simulink model "generic_truck"  (R2025a)
settings: Solver=VariableStepAuto  StartTime=0.0  StopTime=600  FixedStep=0.01  MaxStep=0.001  RelTol=1e-3  EnableMultiTasking=on
libraries: TruckMaker4SL x205, simulink x1
(part 7 of 9)

== matlab function generic_truck/TruckMaker/Subsystem1/ONE_TRACK_MODEL_TRACTOR_UKF/Working Model with 7 measurements ==
  data: z input; u input; xhat output; Q input; R input; Ts input; P output; dxdt output; innovation output; K_out output; S_out output; z_pred_out output; data input
function [xhat, P, dxdt, innovation, K_out, S_out, z_pred_out] = UKF_OneTrack_IMU(z, u, Q, R, Ts,data)

persistent x Pk dxdt_old t p_nom Pp

if isempty(x)
    x = [15;0.1;0.1;7.5;7.5];
end
if isempty(Pk)
    Pk = diag([0.1 0.1 0.1 5 5]);
end
if isempty(dxdt_old)
    dxdt_old = zeros(5,1);
end
if isempty(t)
    t = 0;
end
if isempty(p_nom)
    p_nom = [6800; 12994.917];
    Pp = diag([5000, 20000]).^2;
end

T_sim = 0.001;
t = t + T_sim;
t=data;

if t < 30
    xhat = x;
    P = Pk;
    dxdt = dxdt_old;
    innovation = zeros(length(z),1);
    K_out = zeros(length(x), length(z));
    S_out = eye(length(z));
    z_pred_out = zeros(length(z),1);
    return
end

IDX_VX  = 3; 
IDX_WRL = 6; 
IDX_WRR = 7;

g  = 9.82;

p_cog = [3.473;0;0.925];
p_fax = [4.520;0;0.490];
p_rax = [0.950;0;0.490];
p_imu = [3.600;0;1.000];

lf = abs(p_fax(1)-p_cog(1));
lr = abs(p_cog(1)-p_rax(1));
L  = lf + lr;
h  = p_cog(3);

Rfax = p_fax - p_cog; Rfax(3) = -p_cog(3);
Rrax = p_rax - p_cog; Rrax(3) = -p_cog(3);
Rcog = p_imu - p_cog;

delta = u(1);
T_rl  = u(2);
T_rr  = u(3);
Rwheel = 0.505;
Fx_vehicle = (T_rl + T_rr)/Rwheel;

n  = length(x);
np = length(p_nom);
nSPx = 2*n + 1;
nSPp = 2*np;
nSP  = nSPx + nSPp;

W0 = 1 - (n + np)/3;
Wi = (1 - W0)/(2*(n + np));
gamma = sqrt((n + np)/(1 - W0));

%% ===== STATE SIGMA =====
Pk = (Pk + Pk')/2 + 1e-9*eye(n);
Sx = chol(Pk,'lower');

X = zeros(n,nSPx);
X(:,1) = x;
for i=1:n
    X(:,i+1)   = x + gamma*Sx(:,i);
    X(:,i+1+n) = x - gamma*Sx(:,i);
end

%% ===== PARAM SIGMA =====
Pp = (Pp + Pp')/2 + 1e-9*eye(np);
Sp = chol(Pp,'lower');

SPp = zeros(np,nSPp);
for i=1:np
    SPp(:,i)    = p_nom + gamma*Sp(:,i);
    SPp(:,i+np) = p_nom - gamma*Sp(:,i);
end

%% ===== PREDICTION =====
X_prop = zeros(n,nSP);
dxdt_model = zeros(5,1);

for k=1:nSP
    if k <= nSPx
        Xk = X(:,k); 
        pk = p_nom;
    else
        Xk = x; 
        pk = SPp(:,k-nSPx);
    end

    vx=Xk(1); vy=Xk(2); wz=Xk(3); Cf=Xk(4); Cr=Xk(5);
    m=pk(1); Jz=pk(2);

    v_cog=[vx;vy;0]; omega=[0;0;wz];
    Rotf=[cos(delta) -sin(delta) 0; sin(delta) cos(delta) 0; 0 0 1];

    vf=Rotf.'*(v_cog+cross(omega,Rfax));
    vr=v_cog+cross(omega,Rrax);

    alpha_f=atan2(vf(2),max(abs(vf(1)),0.1));
    alpha_r=atan2(vr(2),max(abs(vr(1)),0.1));

    ax_est=Fx_vehicle/m+vy*wz;

    Ffz=m*g*lr/L - m*ax_est*h/L;
    Frz=m*g*lf/L + m*ax_est*h/L;

    Fy_f=-Cf*alpha_f*Ffz;
    Fy_r=-Cr*alpha_r*Frz;

    dvx=(Fx_vehicle - Fy_f*sin(delta))/m + vy*wz;
    dvy=(Fy_f*cos(delta)+Fy_r)/m - vx*wz;
    dwz=(lf*Fy_f*cos(delta) - lr*Fy_r)/Jz;

    if k==1
        dxdt_model=[dvx;dvy;dwz;0;0];
    end

    X_prop(:,k)=[vx+Ts*dvx; vy+Ts*dvy; wz+Ts*dwz; Cf; Cr];
end

%% ===== MEAN =====
x_pred=zeros(n,1);
for k=1:nSP
    w=(k==1)*W0 + (k>1)*Wi;
    x_pred=x_pred + w*X_prop(:,k);
end

%% ===== COV =====
P_pred=zeros(n);
for k=1:nSPx
    w=(k==1)*W0 + (k>1)*Wi;
    dx=X_prop(:,k)-x_pred;
    P_pred=P_pred + w*(dx*dx');
end
P_pred=P_pred + Q*Ts;

%% ===== NEW SIGMA POINTS =====
P_pred=(P_pred+P_pred')/2 + 1e-9*eye(n);
Sx=chol(P_pred,'lower');

SPx_new=zeros(n,nSPx);
SPx_new(:,1)=x_pred;

for i=1:n
    SPx_new(:,i+1)=x_pred+gamma*Sx(:,i);
    SPx_new(:,i+1+n)=x_pred-gamma*Sx(:,i);
end

%% ===== MEASUREMENT =====
Z=zeros(length(z),nSP);

for k=1:nSP
    if k<=nSPx
        Xk=SPx_new(:,k);
        pk=p_nom;
    else
        Xk=x_pred;
        pk=SPp(:,k-nSPx);
    end

    vx=Xk(1); vy=Xk(2); wz=Xk(3);
    Cf=Xk(4); Cr=Xk(5);

    m=pk(1); Jz=pk(2);

    v_cog=[vx;vy;0]; omega=[0;0;wz];
    Rotf=[cos(delta) -sin(delta) 0; sin(delta) cos(delta) 0; 0 0 1];

    vf=Rotf.'*(v_cog+cross(omega,Rfax));
    vr=v_cog+cross(omega,Rrax);

    alpha_f=atan2(vf(2),max(abs(vf(1)),0.1));
    alpha_r=atan2(vr(2),max(abs(vr(1)),0.1));

    ax_est=Fx_vehicle/m+vy*wz;

    Ffz=m*g*lr/L - m*ax_est*h/L;
    Frz=m*g*lf/L + m*ax_est*h/L;

    Fy_f=-Cf*alpha_f*Ffz;
    Fy_r=-Cr*alpha_r*Frz;

    dvx=(Fx_vehicle - Fy_f*sin(delta))/m;
    dvy=(Fy_f*cos(delta)+Fy_r)/m;
    dwz=(lf*Fy_f*cos(delta) - lr*Fy_r)/Jz;

    a_cog=[dvx;dvy;0];
    alpha_vec=[0;0;dwz];

    a_imu=a_cog + cross(omega,cross(omega,Rcog)) + cross(alpha_vec,Rcog);
    v_imu=v_cog + cross(omega,Rcog);

    omega_rl=vx/Rwheel;
    omega_rr=vx/Rwheel;

    Z(:,k)=[a_imu(1:2); v_imu(1:2); wz; omega_rl; omega_rr];
end

%% ===== z mean =====
z_pred=zeros(length(z),1);
for k=1:nSP
    w=(k==1)*W0 + (k>1)*Wi;
    z_pred=z_pred + w*Z(:,k);
end

%% ===== SENSOR SELECTION =====
valid_idx=true(length(z),1);

if ~isnan(z(IDX_VX))
    valid_idx(IDX_WRL)=false;
    valid_idx(IDX_WRR)=false;
else
    valid_idx(IDX_VX)=false;
end

valid_idx=valid_idx & ~isnan(z);

z_used=z(valid_idx);
z_pred_used=z_pred(valid_idx);
Z_used=Z(valid_idx,:);
R_used=R(valid_idx,valid_idx);

%% ===== S =====
S_cov=zeros(length(z_used));
for k=1:nSP
    w=(k==1)*W0 + (k>1)*Wi;
    dz=Z_used(:,k)-z_pred_used;
    S_cov=S_cov + w*(dz*dz');
end

S_cov=S_cov + R_used;
S_cov=(S_cov+S_cov')/2 + 1e-9*eye(size(S_cov));

%% ===== Pxz =====
Pxz=zeros(n,length(z_used));
for k=1:nSPx
    w=(k==1)*W0 + (k>1)*Wi;
    dx=SPx_new(:,k)-x_pred;
    dz=Z_used(:,k)-z_pred_used;
    Pxz=Pxz + w*(dx*dz');
end

%% ===== UPDATE =====
K=Pxz/S_cov;

x=x_pred + K*(z_used - z_pred_used);
Pk=P_pred - K*S_cov*K';
Pk=(Pk+Pk')/2 + 1e-9*eye(n);

%% ===== OUTPUT =====
xhat=x;
P=Pk;
dxdt=dxdt_model;

innovation=zeros(length(z),1);
innovation(valid_idx)=z_used - z_pred_used;

K_out=zeros(n,length(z));
K_out(:,valid_idx)=K;

S_out=zeros(length(z));
S_out(valid_idx,valid_idx)=S_cov;

z_pred_out=z_pred;

end

== matlab function generic_truck/TruckMaker/Subsystem1/ONE_TRACK_MODEL_TRACTOR_UKF/MATLAB Function1 ==
  data: z input; u input; xhat output; Q input; R input; Ts input; data input; P output; dxdt output; innovation output; K_out output; S_out output; z_pred_out output
function [xhat, P, dxdt, innovation, K_out, S_out, z_pred_out] = UKF_OneTrack_IMU(z, u, Q, R, Ts,data)

persistent x Pk dxdt_old t p_nom Pp

if isempty(x)
    x = [15;0.1;0.1;7.5;7.5];
end
if isempty(Pk)
    Pk = diag([0.1 0.1 0.1 5 5]);
end
if isempty(dxdt_old)
    dxdt_old = zeros(5,1);
end
if isempty(t)
    t = 0;
end
if isempty(p_nom)
    p_nom = [6800; 12994.917];
    Pp = diag([5000, 20000]).^2;
end

T_sim = 0.001;
t = t + T_sim;
t=data;

if t < 30
    xhat = x;
    P = Pk;
    dxdt = dxdt_old;
    innovation = zeros(length(z),1);
    K_out = zeros(length(x), length(z));
    S_out = eye(length(z));
    z_pred_out = zeros(length(z),1);
    return
end

IDX_VX  = 3; 
IDX_WRL = 6; 
IDX_WRR = 7;

g  = 9.82;

p_cog = [3.473;0;0.925];
p_fax = [4.520;0;0.490];
p_rax = [0.950;0;0.490];
p_imu = [3.600;0;1.000];

lf = abs(p_fax(1)-p_cog(1));
lr = abs(p_cog(1)-p_rax(1));
L  = lf + lr;
h  = p_cog(3);

Rfax = p_fax - p_cog; Rfax(3) = -p_cog(3);
Rrax = p_rax - p_cog; Rrax(3) = -p_cog(3);
Rcog = p_imu - p_cog;

delta = u(1);
T_rl  = u(2);
T_rr  = u(3);
Rwheel = 0.505;
Fx_vehicle = (T_rl + T_rr)/Rwheel;

n  = length(x);
np = length(p_nom);
nSPx = 2*n + 1;
nSPp = 2*np;
nSP  = nSPx + nSPp;

W0 = 1 - (n + np)/3;
Wi = (1 - W0)/(2*(n + np));
gamma = sqrt((n + np)/(1 - W0));

%% ===== STATE SIGMA =====
Pk = (Pk + Pk')/2 + 1e-9*eye(n);
Sx = chol(Pk,'lower');

X = zeros(n,nSPx);
X(:,1) = x;
for i=1:n
    X(:,i+1)   = x + gamma*Sx(:,i);
    X(:,i+1+n) = x - gamma*Sx(:,i);
end

%% ===== PARAM SIGMA =====
Pp = (Pp + Pp')/2 + 1e-9*eye(np);
Sp = chol(Pp,'lower');

SPp = zeros(np,nSPp);
for i=1:np
    SPp(:,i)    = p_nom + gamma*Sp(:,i);
    SPp(:,i+np) = p_nom - gamma*Sp(:,i);
end

%% ===== PREDICTION =====
X_prop = zeros(n,nSP);
dxdt_model = zeros(5,1);

for k=1:nSP
    if k <= nSPx
        Xk = X(:,k); 
        pk = p_nom;
    else
        Xk = x; 
        pk = SPp(:,k-nSPx);
    end

    vx=Xk(1); vy=Xk(2); wz=Xk(3); Cf=Xk(4); Cr=Xk(5);
    m=pk(1); Jz=pk(2);

    v_cog=[vx;vy;0]; 
    omega=[0;0;wz];

    Rotf=[cos(delta) -sin(delta) 0;
          sin(delta)  cos(delta)  0; 
           0          0          1];

    vf=Rotf.'*(v_cog+cross(omega,Rfax));
    vr=v_cog+cross(omega,Rrax);

    alpha_f=atan2(vf(2),max(abs(vf(1)),0.1));
    alpha_r=atan2(vr(2),max(abs(vr(1)),0.1));

    ax_est=Fx_vehicle/m+vy*wz;

    Ffz=m*g*lr/L - m*ax_est*h/L;
    Frz=m*g*lf/L + m*ax_est*h/L;

    Fy_f=-Cf*alpha_f*Ffz;
    Fy_r=-Cr*alpha_r*Frz;

    dvx=(Fx_vehicle - Fy_f*sin(delta))/m + vy*wz;
    dvy=(Fy_f*cos(delta)+Fy_r)/m - vx*wz;
    dwz=(lf*Fy_f*cos(delta) - lr*Fy_r)/Jz;

    if k==1
        dxdt_model=[dvx;dvy;dwz;0;0];
    end

    X_prop(:,k)=[vx+Ts*dvx; vy+Ts*dvy; wz+Ts*dwz; Cf; Cr];
end

%% ===== MEAN =====
x_pred=zeros(n,1);
for k=1:nSP
    w=(k==1)*W0 + (k>1)*Wi;
    x_pred=x_pred + w*X_prop(:,k);
end

%% ===== COV =====
P_pred=zeros(n);
for k=1:nSPx
    w=(k==1)*W0 + (k>1)*Wi;
    dx=X_prop(:,k)-x_pred;
    P_pred=P_pred + w*(dx*dx');
end
P_pred=P_pred + Q*Ts;

%% ===== NEW SIGMA POINTS =====
P_pred=(P_pred+P_pred')/2 + 1e-9*eye(n);
Sx=chol(P_pred,'lower');

SPx_new=zeros(n,nSPx);
SPx_new(:,1)=x_pred;

for i=1:n
    SPx_new(:,i+1)  =x_pred+gamma*Sx(:,i);
    SPx_new(:,i+1+n) =x_pred-gamma*Sx(:,i);
end

%% ===== MEASUREMENT =====
Z=zeros(length(z),nSP);

for k=1:nSP
    if k<=nSPx
        Xk=SPx_new(:,k);
        pk=p_nom;
    else
        Xk=x_pred;
        pk=SPp(:,k-nSPx);
    end

    vx=Xk(1); vy=Xk(2); wz=Xk(3);
    Cf=Xk(4); Cr=Xk(5);

    m=pk(1); Jz=pk(2);

    v_cog=[vx;vy;0]; omega=[0;0;wz];
    Rotf=[cos(delta) -sin(delta) 0; sin(delta) cos(delta) 0; 0 0 1];

    vf=Rotf.'*(v_cog+cross(omega,Rfax));
    vr=v_cog+cross(omega,Rrax);

    alpha_f=atan2(vf(2),max(abs(vf(1)),0.1));
    alpha_r=atan2(vr(2),max(abs(vr(1)),0.1));

    ax_est=Fx_vehicle/m+vy*wz;

    Ffz=m*g*lr/L - m*ax_est*h/L;
    Frz=m*g*lf/L + m*ax_est*h/L;

    Fy_f=-Cf*alpha_f*Ffz;
    Fy_r=-Cr*alpha_r*Frz;

    dvx=(Fx_vehicle - Fy_f*sin(delta))/m;
    dvy=(Fy_f*cos(delta)+Fy_r)/m;
    dwz=(lf*Fy_f*cos(delta) - lr*Fy_r)/Jz;

    a_cog=[dvx;dvy;0];
    alpha_vec=[0;0;dwz];

    a_imu=a_cog + cross(omega,cross(omega,Rcog)) + cross(alpha_vec,Rcog);
    v_imu=v_cog + cross(omega,Rcog);

    omega_rl=vx/Rwheel;
    omega_rr=vx/Rwheel;

    Z(:,k)=[a_imu(1:2); v_imu(1:2); wz; omega_rl; omega_rr];
end

%% ===== z mean =====
z_pred=zeros(length(z),1);
for k=1:nSP
    w=(k==1)*W0 + (k>1)*Wi;
    z_pred=z_pred + w*Z(:,k);
end

%% ===== SENSOR SELECTION =====
valid_idx=true(length(z),1);

if ~isnan(z(IDX_VX))
    valid_idx(IDX_WRL)=false;
    valid_idx(IDX_WRR)=false;
else
    valid_idx(IDX_VX)=false;
end

valid_idx=valid_idx & ~isnan(z);

z_used=z(valid_idx);
z_pred_used=z_pred(valid_idx);
Z_used=Z(valid_idx,:);
R_used=R(valid_idx,valid_idx);

%% ===== S =====
S_cov=zeros(length(z_used));
for k=1:nSP
    w=(k==1)*W0 + (k>1)*Wi;
    dz=Z_used(:,k)-z_pred_used;
    S_cov=S_cov + w*(dz*dz');
end

S_cov=S_cov + R_used;
S_cov=(S_cov+S_cov')/2 + 1e-9*eye(size(S_cov));

%% ===== Pxz =====
Pxz=zeros(n,length(z_used));
for k=1:nSPx
    w=(k==1)*W0 + (k>1)*Wi;
    dx=SPx_new(:,k)-x_pred;
    dz=Z_used(:,k)-z_pred_used;
    Pxz=Pxz + w*(dx*dz');
end

%% ===== UPDATE =====
K=Pxz/S_cov;

x=x_pred + K*(z_used - z_pred_used);
Pk=P_pred - K*S_cov*K';
Pk=(Pk+Pk')/2 + 1e-9*eye(n);

%% ===== OUTPUT =====
xhat=x;
P=Pk;
dxdt=dxdt_model;

innovation=zeros(length(z),1);
innovation(valid_idx)=z_used - z_pred_used;

K_out=zeros(n,length(z));
K_out(:,valid_idx)=K;

S_out=zeros(length(z));
S_out(valid_idx,valid_idx)=S_cov;

z_pred_out=z_pred;

end

== matlab function generic_truck/TruckMaker/Subsystem1/ONE_TRACK_MODEL_TRACTOR_UKF/MATLAB Function2 ==
  data: z input; u input; Q input; R input; Ts input; xhat output; data input; P output; dxdt output; innovation output; K_out output; S_out output; z_pred_out output
function [xhat, P, dxdt, innovation, K_out, S_out, z_pred_out] = UKF_OneTrack_IMU(z, u, Q, R, Ts, data)

persistent x Pk dxdt_old t

%% =========================
%% INIT
%% =========================
if isempty(x)
    % [vx vy wz Cf Cr bax]
    x = [15;0.1;0.1;7.5;7.5;0];
end

if isempty(Pk)
    Pk = diag([0.1 0.1 0.1 5 5 0.5]);
end

if isempty(dxdt_old)
    dxdt_old = zeros(6,1);
end

if isempty(t)
    t = 0;
end

t = data;

if t < 30
    xhat = x;
    P = Pk;
    dxdt = dxdt_old;
    innovation = zeros(length(z),1);
    K_out = zeros(length(x), length(z));
    S_out = eye(length(z));
    z_pred_out = zeros(length(z),1);
    return
end

IDX_VX = 3;
IDX_VY = 4;

%% =========================
%% VEHICLE CONSTANTS
%% =========================
g  = 9.82;

p_cog = [3.473;0;0.925];
p_fax = [4.520;0;0.490];
p_rax = [0.950;0;0.490];
p_imu = [3.600;0;1.000];

lf = abs(p_fax(1)-p_cog(1));
lr = abs(p_cog(1)-p_rax(1));
L  = lf + lr;
h  = p_cog(3);

Rfax = p_fax - p_cog; Rfax(3) = -p_cog(3);
Rrax = p_rax - p_cog; Rrax(3) = -p_cog(3);
Rcog = p_imu - p_cog;

%% =========================
%% INPUTS
%% =========================
delta = u(1);
T_rl  = u(2);
T_rr  = u(3);
Rwheel = 0.505;
Fx_vehicle = (T_rl + T_rr)/Rwheel;

%% =========================
%% UKF PARAMS
%% =========================
n = length(x);
nSPx = 2*n + 1;

W0 = 1 - n/3;
Wi = (1 - W0)/(2*n);
gamma = sqrt(n/(1-W0));

%% =========================
%% SIGMA POINTS (PRIOR)
%% =========================
Pk = (Pk + Pk')/2 + 1e-9*eye(n);
Sx = chol(Pk,'lower');

X_pre = zeros(n,nSPx);
X_pre(:,1) = x;

for i=1:n
    X_pre(:,i+1)   = x + gamma*Sx(:,i);
    X_pre(:,i+1+n) = x - gamma*Sx(:,i);
end

%% =========================
%% PREDICTION
%% =========================
X_pred = zeros(n,nSPx);
dxdt_model = zeros(n,1);

m = 6800; 
Jz = 12994.917;

for k=1:nSPx

    Xk = X_pre(:,k);

    vx = Xk(1); vy = Xk(2); wz = Xk(3);
    Cf = Xk(4); Cr = Xk(5);
    bax = Xk(6);

    v_cog = [vx; vy; 0]; 
    omega = [0; 0; wz];

    Rotf = [cos(delta) -sin(delta) 0;
            sin(delta)  cos(delta) 0;
            0 0 1];

    vf = Rotf.'*(v_cog + cross(omega,Rfax));
    vr = v_cog + cross(omega,Rrax);

    alpha_f = atan2(vf(2), max(abs(vf(1)),0.1));
    alpha_r = atan2(vr(2), max(abs(vr(1)),0.1));

    ax_est = Fx_vehicle/m + vy*wz;

    Ffz = m*g*lr/L - m*ax_est*h/L;
    Frz = m*g*lf/L + m*ax_est*h/L;

    Fy_f = -Cf*alpha_f*Ffz;
    Fy_r = -Cr*alpha_r*Frz;

    dvx = (Fx_vehicle - Fy_f*sin(delta))/m + vy*wz;

    % Testa DÄMPNING här (NYCKELN!)
    dvy = (Fy_f*cos(delta)+Fy_r)/m - vx*wz;

    dwz = (lf*Fy_f*cos(delta) - lr*Fy_r)/Jz;

    if k==1
        dxdt_model = [dvx; dvy; dwz; 0; 0; 0];
    end

    X_pred(:,k) = [
        vx + Ts*dvx
        vy + Ts*dvy
        wz + Ts*dwz
        Cf
        Cr
        bax
    ];
end

%% =========================
%% MEAN
%% =========================
x_pred = zeros(n,1);
for k=1:nSPx
    w = (k==1)*W0 + (k>1)*Wi;
    x_pred = x_pred + w*X_pred(:,k);
end

%% =========================
%% COVARIANCE
%% =========================
P_pred = zeros(n);
for k=1:nSPx
    w = (k==1)*W0 + (k>1)*Wi;
    dx = X_pred(:,k) - x_pred;
    P_pred = P_pred + w*(dx*dx');
end

P_pred = P_pred + Q*Ts;
P_pred = (P_pred + P_pred')/2 + 1e-9*eye(n);

%% =========================
%% SIGMA POINTS (POST)
%% =========================
Sx = chol(P_pred,'lower');

X_post = zeros(n,nSPx);
X_post(:,1) = x_pred;

for i=1:n
    X_post(:,i+1)   = x_pred + gamma*Sx(:,i);
    X_post(:,i+1+n) = x_pred - gamma*Sx(:,i);
end

%% =========================
%% MEASUREMENT MODEL
%% =========================
Z = zeros(length(z), nSPx);

for k=1:nSPx

    Xk = X_post(:,k);

    vx = Xk(1); vy = Xk(2); wz = Xk(3);
    Cf = Xk(4); Cr = Xk(5);
    bax = Xk(6);

    v_cog = [vx; vy; 0]; 
    omega=[0;0;wz];

    Rotf=[cos(delta) -sin(delta) 0;
          sin(delta)  cos(delta) 0;
          0 0 1];

    vf = Rotf.'*(v_cog+cross(omega,Rfax));
    vr = v_cog+cross(omega,Rrax);

    alpha_f = atan2(vf(2), max(abs(vf(1)),0.1));
    alpha_r = atan2(vr(2), max(abs(vr(1)),0.1));

    ax_est = Fx_vehicle/m + vy*wz;

    Ffz = m*g*lr/L - m*ax_est*h/L;
    Frz = m*g*lf/L + m*ax_est*h/L;

    Fy_f = -Cf*alpha_f*Ffz;
    Fy_r = -Cr*alpha_r*Frz;
    
    dvx = (Fx_vehicle - Fy_f*sin(delta))/m;
    dvy = (Fy_f*cos(delta)+Fy_r)/m;
    dwz = (lf*Fy_f*cos(delta) - lr*Fy_r)/Jz;

    a_cog = [dvx; dvy; 0];
    alpha_vec=[0;0;dwz];

    a_imu = a_cog + cross(omega,cross(omega,Rcog)) + cross(alpha_vec,Rcog);
    v_imu = v_cog + cross(omega,Rcog);

    ax_meas = a_imu(1) + bax;

    Z(:,k) = [
        ax_meas
        a_imu(2)
        v_imu(1:2)
        wz
    ];
end

%% =========================
%% MEASUREMENT MEAN
%% =========================
z_pred = zeros(length(z),1);
for k=1:nSPx
    w = (k==1)*W0 + (k>1)*Wi;
    z_pred = z_pred + w*Z(:,k);
end

%% =========================
%% SENSOR SELECTION
%% =========================
valid_idx = true(length(z),1);

if isnan(z(IDX_VX))
    valid_idx(IDX_VX) = false;
    valid_idx(IDX_VY) = false;
end

valid_idx = valid_idx & ~isnan(z);

z_used = z(valid_idx);
z_pred_used = z_pred(valid_idx);
Z_used = Z(valid_idx,:);
R_used = R(valid_idx,valid_idx);

%% =========================
%% S + Pxz
%% =========================
S_cov = zeros(length(z_used));
Pxz = zeros(n,length(z_used));

for k=1:nSPx
    w = (k==1)*W0 + (k>1)*Wi;

    dz = Z_used(:,k)-z_pred_used;
    dx = X_post(:,k)-x_pred;

    S_cov = S_cov + w*(dz*dz');
    Pxz = Pxz + w*(dx*dz');
end

S_cov = S_cov + R_used;
S_cov = (S_cov + S_cov')/2 + 1e-9*eye(size(S_cov));

%% =========================
%% UPDATE
%% =========================
K = Pxz / S_cov;

x = x_pred + K*(z_used - z_pred_used);
Pk = P_pred - K*S_cov*K';
Pk = (Pk + Pk')/2 + 1e-9*eye(n);

%% =========================
%% OUTPUT
%% =========================
xhat = x;
P = Pk;
dxdt = dxdt_model;

innovation = zeros(length(z),1);
innovation(valid_idx) = z_used - z_pred_used;

K_out = zeros(n,length(z));
K_out(:,valid_idx) = K;

S_out = zeros(length(z));
S_out(valid_idx,valid_idx) = S_cov;

z_pred_out = z_pred;

end

== matlab function generic_truck/TruckMaker/Subsystem1/Subsystem_Noisey Measurements/MATLAB Function3 ==
  data: truth input; vel_meas output
function vel_meas = imu_vel_noise(truth)
    

sigma = 0.05; % m/s^2 (tune later)

vel_meas = truth + sigma * randn(size(truth));


end

== matlab function generic_truck/TruckMaker/Subsystem1/ONE_TRACK_MODEL_TRACTOR_UKF/Included_trailer  ==
  data: z input; u input; xhat output; Q input; R input; Ts input; data input; P output; dxdt output; innovation output; K_out output; S_out output; z_pred_out output
function [xhat, P, dxdt, innovation, K_out, S_out, z_pred_out] = UKF_TruckTrailer(z,u,Q,R,Ts,data)

persistent x Pk dxdt_old t

%% =========================
%% INIT
%% =========================
if isempty(x)
    x = [15;0.1;0.1;7.5;7.5;0;0;6]; % [vx vy wz Cf Cr psi wz_tr Cr_tr]
end

if isempty(Pk)
    Pk = diag([0.1 0.1 0.1 5 5 0.1 0.1 5]);
end

if isempty(dxdt_old)
    dxdt_old = zeros(8,1);
end

if isempty(t)
    t = 0;
end
t = data;

if t < 30
    xhat=x; P=Pk; dxdt=dxdt_old;
    
    innovation=zeros(length(z),1);
    K_out=zeros(length(x), length(z));
    S_out=eye(length(z));
    z_pred_out=zeros(length(z),1);
    return
end

%% =========================
%% CONSTANTS
%% =========================
g = 9.82;

% Truck
m = 6800; Jz = 12994.917; Rwheel = 0.49;

% Trailer
m_tr = 31960; Jz_tr = 145971.764;

% Geometry &  koordinat punkter på Truck
p_cog = [3.473;0;0.925];
p_fax = [4.520;0;0.490];
p_rax = [0.950;0;0.490];
p_imu = [3.600;0;1.000];
hitch = [1.9;0;1.21];

Rcog = p_imu - p_cog;



% Geometry Trailer
p_cog_tr = [-6.195;0;1.95];
p_rax_tr = [-9.0;0;0.490];
hitch_tr = [-1.25;0;1.25];

lf = abs(p_fax(1)-p_cog(1)); 
lr = abs(p_cog(1)-p_rax(1)); 
L = lf + lr;

h = p_cog(3);

Rfax = p_fax - p_cog; Rfax(3)=-p_cog(3);
Rrax = p_rax - p_cog; Rrax(3)=-p_cog(3);

Rhitch = hitch - p_cog;
lhitch = Rhitch(1);

lfhitch = abs(p_fax(1) -hitch(1)); 

lf_tr = abs(hitch_tr(1)-p_cog_tr(1));
lr_tr = abs(p_cog_tr(1)-p_rax_tr(1));
L_tr = lf_tr + lr_tr;
h_tr = p_cog_tr(3);
hHitch= hitch(3);

Rrax_tr = p_rax_tr - hitch_tr; Rrax_tr(3)=-hitch_tr(3);

%% =========================
%% INPUTS
%% =========================
delta = u(1); % steering to raod angle 

% Rear wheel driv
T_rl = u(2);   
T_rr = u(3);

Fxh = u(4); % Inertial Frame  
Fyh = u(5); % Inertial Frame 

Fx_vehicle = (T_rl+T_rr)/Rwheel;

%% =========================
%% UKF PARAMS
%% =========================
n = length(x);
nSPx = 2*n+1;

W0 = 1 - n/3;
Wi = (1 - W0)/(2*n);
gamma = sqrt(n/(1 - W0));

%% =========================
%% SIGMA POINTS (PRIOR)
%% =========================
Pk = (Pk+Pk')/2 + 1e-9*eye(n);
Sx = chol(Pk,'lower');

X_pre = zeros(n,nSPx);
X_pre(:,1) = x;

for i=1:n
    X_pre(:,i+1)   = x + gamma*Sx(:,i);
    X_pre(:,i+1+n) = x - gamma*Sx(:,i);
end

%% =========================
%% PREDICTION
%% =========================
X_pred = zeros(n,nSPx);
dxdt_model = zeros(n,1);

for k=1:nSPx

    Xk = X_pre(:,k);
    % Traktor CoG
    vx=Xk(1); vy=Xk(2); wz=Xk(3);
    Cf=Xk(4); Cr=Xk(5);
    
    %Trialer 
    psi=Xk(6); wz_tr=Xk(7); Cr_tr=Xk(8);

    v_cog=[vx;vy;0];
    omega=[0;0;wz];

    %% ===== TRAILER =====
    v_hitch_truck = v_cog + cross(omega,Rhitch);

    Rot_tr=[cos(psi) -sin(psi) 0;
            sin(psi)  cos(psi) 0;
            0 0 1];

    omega_tr=[0;0;wz_tr];

    v_hitch_trailer = -Rot_tr.' * v_hitch_truck;
    
    % velocity of trailer wheel at rear axle contact point  
    v_tr_ax = v_hitch_trailer + cross(omega_tr,Rrax_tr);
    
    % slip
    alpha_tr = atan2(v_tr_ax(2),max(abs(v_tr_ax(1)),0.1));
    
    % load transfer approximation 
    ax_tr = Fxh/m_tr;
    
    Fz_hitch = m_tr*g*lr_tr/L_tr + m_tr*ax_tr*(h_tr-hHitch)/L_tr;
    Fz_tr    = m_tr*g - Fz_hitch;
    
    %Brush Model 
    Fy_tr = -Cr_tr*alpha_tr*Fz_tr;

    %% ===== TRUCK =====
    %Rotation Matris 
    Rotf=[cos(delta) -sin(delta) 0;
          sin(delta)  cos(delta) 0;
          0                0     1];
    
    % velocities at contact point 
    vf = Rotf.'*(v_cog + cross(omega,Rfax));
    vr = v_cog + cross(omega,Rrax);
    
    %slip per wheel 
    alpha_f = atan2(vf(2),max(abs(vf(1)),0.1));
    alpha_r = atan2(vr(2),max(abs(vr(1)),0.1));
    
    F_hitch_trailer=[u(4);u(5);0];

    F_hitch_body= Rot_tr * F_hitch_trailer;

    % load transfer approximation
    ax_est = (Fx_vehicle + F_hitch_body(1))/m + vy*wz;

    %Ffz = m*g*lr/L - m*ax_est*(h-hHitch)/L + Fz_hitch*(L-lfhitch)/L - F_hitch_body(1)*hHitch/L;
    %Frz = m*g*lf/L + m*ax_est*(h-hHitch)/L;
    
      Ffz = m*g*lr/L + m*ax_est*(h)/L  + Fz_hitch;
      Frz= m*g*lf/L - Ffz ;

    %brsuh model 
    Fy_f = -Cf*alpha_f*Ffz;
    Fy_r = -Cr*alpha_r*Frz;


    %% ===== DYNAMICS =====
    %dvx = (Fx_vehicle - Fy_f*sin(delta) - Fxh*cos(psi) + Fyh*sin(psi))/m + vy*wz;
    dvx = (Fx_vehicle - Fy_f*sin(delta) - F_hitch_body(1))/m + vy*wz;

    %dvy = (Fy_f*cos(delta)+Fy_r - Fyh*cos(psi) - Fxh*sin(psi))/m - vx*wz;
    dvy = (Fy_f*cos(delta) + Fy_r - F_hitch_body(2))/m - vx*wz;
    
    dwz = (lf*Fy_f*cos(delta)-lr*Fy_r)/Jz;% - lhitch*(Fyh*cos(psi) + Fxh*sin(psi)))/Jz;
    %dwz = (lf*Fy_f*cos(delta) -lr*Fy_r - lhitch*(F_hitch_body(2)))/Jz;
    
    dpsi = wz_tr - wz; % Articulation angle 

    dwz_tr = (lr_tr*Fy_tr - lf_tr*Fyh)/Jz_tr;

    if k==1
        dxdt_model=[dvx;dvy;dwz;0;0;dpsi;dwz_tr;0];
    end

    X_pred(:,k) = Xk + Ts*[dvx;
                           dvy;
                           dwz;
                           0;
                           0;
                           dpsi;
                           dwz_tr;
                           0];
end

%% ===== MEAN & COV
x_pred=zeros(n,1);
P_pred=zeros(n);

for k=1:nSPx
    w=(k==1)*W0+(k>1)*Wi;
    x_pred=x_pred+w*X_pred(:,k);
end

for k=1:nSPx
    w=(k==1)*W0+(k>1)*Wi;
    dx=X_pred(:,k)-x_pred;
    P_pred=P_pred+w*(dx*dx');
end

P_pred=P_pred+Q*Ts;
P_pred=(P_pred+P_pred')/2 + 1e-9*eye(n);

%% =========================
%% MEASUREMENT
%% =========================
Sx=chol(P_pred,'lower');

X_post=zeros(n,nSPx);
X_post(:,1)=x_pred;

for i=1:n
    X_post(:,i+1)  =x_pred + gamma*Sx(:,i);
    X_post(:,i+1+n)=x_pred - gamma*Sx(:,i);
end

Z=zeros(length(z),nSPx);

for k=1:nSPx

    Xk=X_post(:,k);

   % Traktor CoG
    vx=Xk(1); vy=Xk(2); wz=Xk(3);
    Cf=Xk(4); Cr=Xk(5);
    
    %Trialer 
    psi=Xk(6); wz_tr=Xk(7); Cr_tr=Xk(8); 
    
    v_cog=[vx;vy;0];
    omega=[0;0;wz];

    %% ===== TRAILER =====
    v_hitch_truck = v_cog + cross(omega,Rhitch);

    Rot_tr=[cos(psi) -sin(psi) 0;
            sin(psi)  cos(psi) 0;
            0 0 1];

    omega_tr=[0;0;wz_tr];

    v_hitch_trailer = Rot_tr.' * v_hitch_truck;
    
    % velocity of trailer wheel at rear axle contact point  
    v_tr_ax = v_hitch_trailer + cross(omega_tr,Rrax_tr);
    
    % slip
    alpha_tr = atan2(v_tr_ax(2),max(abs(v_tr_ax(1)),0.1));
    
    % load transfer approximation 
    ax_tr = (Fxh) / m_tr; % misstänker att vi kan ha ett fel här 
    
    Fz_hitch = m_tr*g*lr_tr/L_tr + m_tr*ax_tr*(h_tr-hHitch)/L_tr;
    Fz_tr = m_tr*g - Fz_hitch;
    
    %Brush Model 
    Fy_tr = -Cr_tr*alpha_tr*Fz_tr;

    %% ===== TRUCK =====    
    %Rotation Matris 
    Rotf=[cos(delta) -sin(delta) 0;
          sin(delta)  cos(delta) 0;
          0                0     1];
    
    % velocities at contact point 
    vf = Rotf.'*(v_cog + cross(omega,Rfax));
    vr = v_cog + cross(omega,Rrax);
    
    %slip per wheel 
    alpha_f = atan2(vf(2),max(abs(vf(1)),0.1));
    alpha_r = atan2(vr(2),max(abs(vr(1)),0.1));
    
    F_hitch_trailer=[u(4);u(5);0];

    F_hitch_body= Rot_tr* F_hitch_trailer;

    % load transfer approximation
    ax_est = (Fx_vehicle + F_hitch_body(1))/m + vy*wz;

    %Ffz = m*g*lr/L - m*ax_est*(h)/L + Fz_hitch*(L-lfhitch)/L - F_hitch_body(1)*hHitch/L;
    %Frz = m*g*lf/L + m*ax_est*(h-hHitch)/L;

      Ffz = m*g*lr/L + m*ax_est*(h)/L  + Fz_hitch;
      Frz= m*g*lf/L - Ffz ;

    %brsuh model 
    Fy_f = -Cf*alpha_f*Ffz;
    Fy_r = -Cr*alpha_r*Frz;


    %% ===== DYNAMICS =====
    %dvx = (Fx_vehicle - Fy_f*sin(delta) - Fxh*cos(psi) + Fyh*sin(psi))/m + vy*wz;
    dvx = (Fx_vehicle - Fy_f*sin(delta) - F_hitch_body(1))/m ;

    %dvy = (Fy_f*cos(delta)+Fy_r - Fyh*cos(psi) - Fxh*sin(psi))/m - vx*wz;
    dvy = (Fy_f*cos(delta)+ Fy_r - F_hitch_body(2))/m;
    
    dwz = (lf*Fy_f*cos(delta)-lr*Fy_r)/Jz;%  - lhitch*(Fyh*cos(psi) + Fxh*sin(psi)))/Jz;
    %dwz = (lf*Fy_f*cos(delta) -lr*Fy_r - lhitch*(F_hitch_body(2)))/Jz;
    
    dpsi = wz_tr - wz; % Articulation angle 

    dwz_tr = (lr_tr*Fy_tr - lf_tr*Fyh )/Jz_tr;

    a_cog=[dvx;dvy;0];
    alpha_vec=[0;0;dwz];

    a_imu=a_cog + cross(omega,cross(omega,Rcog)) + cross(alpha_vec,Rcog);
    v_imu=v_cog + cross(omega,Rcog);

    omega_rl=vx/Rwheel;
    omega_rr=vx/Rwheel;

    omega_tr_ML= v_tr_ax(1)/Rwheel;
    omega_tr_MR= v_tr_ax(1)/Rwheel;

    Z(:,k)=[a_imu(1:2); v_imu(1);v_imu(2); wz; omega_rl; omega_rr; omega_tr_ML; omega_tr_MR];
end

%% ===== REST (sensor selection + update) = DIN ORIGINAL
z_pred=zeros(length(z),1);
for k=1:nSPx
    w=(k==1)*W0+(k>1)*Wi;
    z_pred=z_pred+w*Z(:,k);
end

valid_idx=true(length(z),1);
valid_idx=valid_idx & ~isnan(z);

z_used=z(valid_idx);
z_pred_used=z_pred(valid_idx);
Z_used=Z(valid_idx,:);
R_used=R(valid_idx,valid_idx);

S_cov=zeros(length(z_used));
Pxz=zeros(n,length(z_used));

for k=1:nSPx
    w=(k==1)*W0+(k>1)*Wi;
    dz=Z_used(:,k)-z_pred_used;
    dx=X_post(:,k)-x_pred;
    S_cov=S_cov+w*(dz*dz');
    Pxz=Pxz+w*(dx*dz');
end

S_cov=S_cov+R_used;
S_cov=(S_cov+S_cov')/2 + 1e-9*eye(size(S_cov));

K=Pxz/S_cov;

x=x_pred + K*(z_used - z_pred_used);
Pk=P_pred - K*S_cov*K';
Pk=(Pk+Pk')/2 + 1e-9*eye(n);

%% OUTPUT
xhat=x;
P=Pk;
dxdt=dxdt_model;

innovation=zeros(length(z),1);
innovation(valid_idx)=z_used - z_pred_used;

K_out=zeros(n,length(z));
K_out(:,valid_idx)=K;

S_out=zeros(length(z));
S_out(valid_idx,valid_idx)=S_cov;

z_pred_out=z_pred;

end

== matlab function generic_truck/TruckMaker/Tractor_Subsystem /EKF_ONE_TRACK ==
  data: z input; u input; xhat output; Q input; R input; Ts input; P output
function [xhat, P] = EKF_Bicycle_Full_NoBias(z, u, Q, R, Ts)
% EKF for One-Track / Bicycle Model (No IMU Bias)
% States: x = [vx; vy; r; Cf; Cr]
% Measurements: z = [ax; ay; vx; vy; r; wL; wR]

%% ---------------- Persistent safe initialization ----------------
persistent x Pk initialized

% Säker initialisering
if isempty(x)
    x = [15; 0; 0.05; 2e4; 2e4];  % vx, vy, r, Cf, Cr
end

if isempty(Pk)
    Pk = diag([1 1 0.05 4e4 4e4].^2); % 5x5
end

if isempty(initialized)
    initialized = true;
end


%% ---------------- Vehicle parameters ----------------

m  = 6800;        %  mass
g  = 9.82;        % gravity contanst   
Jz = 12994.917;   % yaw interia
Rw = 0.49;          % wheel radius
width = 2.49;       % track width

p_cog  = [3.473; 0; 0.925];
p_fax  = [4.520; 0; 0.490];

p_rax  = [0.950; 0; 0.490];
p_imu  = [3.600; 0; 1.000];

lf = abs(p_fax(1)-p_cog(1));   % front CoG distance
lr = abs(p_cog(1)-p_rax(1));   % rear CoG distance
L  = lf + lr;
h  = p_cog(3);

Rfax = p_fax - p_imu; Rfax(3) = -p_imu(3);
Rrax = p_rax - p_imu; Rrax(3) = -p_imu(3);
Rcog = p_cog - p_imu;

%% ---------------- Inputs ----------------
delta = u(1);                             % Average steering Angle (FL +FR)/2
T_rl  = u(2);                             % torque RL  
T_rr  = u(3);                             %torque RR
Rwheel = 0.49;                            % wheel radius
Fx_vehicle = (T_rl + T_rr)/Rwheel;        % longitudinal force

%% ---------------- States ----------------
vx = x(1); vy = x(2); r = x(3); Cf = x(4); Cr= x(5);

Rotf = [ cos(delta)     -sin(delta)     0;
         sin(delta)      cos(delta)     0;
             0              0           1];

v_cog = [vx; vy; 0];
omega = [0;0;r];

% Contact patch velocities
vf = Rotf.' * (v_cog + cross(omega,Rfax));
vr = v_cog + cross(omega,Rrax);

alpha_f = atan2(vf(2), max(abs(vf(1)),0.1));
alpha_r = atan2(vr(2), max(abs(vr(1)),0.1));

% Longitudinal accel estimate to compute the vertikel forces
dvx_temp = Fx_vehicle/m + vy*r;

% Normal forces
Ffz = m*g*lr/L - m*dvx_temp*h/L;
Frz = m*g*lf/L + m*dvx_temp*h/L;

% Tire forces
Fy_f = Cf * alpha_f * Ffz;
Fy_r = Cr * alpha_r * Frz;

% Full dynamics 
dvx = (Fx_vehicle - Fy_f*sin(delta))/m + vy*r;
dvy = (Fy_f*cos(delta) + Fy_r)/m - vx*r;
dr  = (lf*Fy_f*cos(delta) - lr*Fy_r)/Jz;

% State propagation
xdot = [dvx; dvy; dr; 0; 0];
x_pred = x + Ts*xdot;

%% ---------------- Jacobian F ----------------
F= zeros(5,5);
F(1,:) = [                                1 - (Cf*Ts*sin(delta)*(vy + lf*r))/(m*vx^2),              Ts*(r + (Cf*sin(delta))/(m*vx)),                   Ts*(vy + (Cf*lf*sin(delta))/(m*vx)),    -(Ts*sin(delta)*(delta - (vy + lf*r)/vx))/m,                            0];
F(2,:) = [  -Ts*(r - ((Cr*(vy - lr*r))/vx^2 + (Cf*cos(delta)*(vy + lf*r))/vx^2)/m),      1 - (Ts*(Cr/vx + (Cf*cos(delta))/vx))/m,    -Ts*(vx - ((Cr*lr)/vx - (Cf*lf*cos(delta))/vx)/m),     (Ts*cos(delta)*(delta - (vy + lf*r)/vx))/m,    -(Ts*(vy - lr*r))/(m*vx)];
F(3,:) = [-(Ts*((Cr*lr*(vy - lr*r))/vx^2 - (Cf*lf*cos(delta)*(vy + lf*r))/vx^2))/Jz, (Ts*((Cr*lr)/vx - (Cf*lf*cos(delta))/vx))/Jz, 1 - (Ts*((Cf*cos(delta)*lf^2)/vx + (Cr*lr^2)/vx))/Jz, (Ts*lf*cos(delta)*(delta - (vy + lf*r)/vx))/Jz, (Ts*lr*(vy - lr*r))/(Jz*vx)];
F(4,:) = [                                                                            0,                                              0,                                                      0,                                                 1,                            0];
F(5,:) = [                                                                            0,                                              0,                                                      0,                                                 0,                            1];


%% ---------------- Covariance prediction ----------------
P_pred = F*Pk*F' + Q;

%% ---------------- Measurement model ----------------
ax_hat = dvx -  vy*r;                % longitudinal accel
ay_hat = dvy + vx*r;                % lateral accel
%vx_hat = vx;
%vy_hat = vy;
%r_hat  = r;
%wL_hat = (vx - width/2 * r)/Rw;
%wR_hat = (vx + width/2 * r)/Rw;

a_cog = [ax_hat; ay_hat; 0];
alpha_vec = [0;0;dr];

% Transform to IMU
a_imu = a_cog - cross(omega, cross(omega,Rcog))- cross(alpha_vec,Rcog);
v_imu = v_cog + cross(omega,Rcog);

z_hat = [a_imu(1:2);
         v_imu(1:2);
         alpha_vec(3);
         omega(3)];

%z_hat = [ax_hat; ay_hat; vx_hat; vy_hat; dr_hat r_hat; wL_hat; wR_hat];

%% ---------------- Measurement Jacobian H ----------------
H = zeros(size(z_hat,1),size(x,1));

%H = zeros(7,5);
H(1,:) = [                               1 - (Cf*Ts*sin(delta)*(vy + lf*r))/(m*vx^2),         Ts*(r + (Cf*sin(delta))/(m*vx)) - r,                      Ts*(vy + (Cf*lf*sin(delta))/(m*vx)) - vy, -(Ts*sin(delta)*(delta - (vy + lf*r)/vx))/m,                            0];
H(2,:) = [-Ts*(r - ((Cr*(vy - lr*r))/vx^2 + (Cf*cos(delta)*(vy + lf*r))/vx^2)/m), 1 - (Ts*(Cr/vx + (Cf*cos(delta))/vx))/m, vx - Ts*(vx - ((Cr*lr)/vx - (Cf*lf*cos(delta))/vx)/m),  (Ts*cos(delta)*(delta - (vy + lf*r)/vx))/m, -(Ts*(vy - lr*r))/(m*vx)];
H(3,:) = [                                                                             1,                                               0,                                                                 0,                                               0,            0];
H(4,:) = [                                                                             0,                                               1,                                                                 0,                                               0,            0];
H(5,:) = [                                                                             0,                                               0,                                                                 0,                                               0,            0];
H(6,:) = [                                                                             0,                                               0,                                                                 1,                                               0,            0];
%H(7,:) = [                                                                             1/Rw,                                            0,                                                     -width/(2*Rw),                                               0,            0];
%H(8,:) = [                                                                             1/Rw,                                            0,                                                      width/(2*Rw),                                               0,            0];

%% ---------------- EKF update ----------------
S = H*P_pred*H' + R;
K = P_pred*H'/(S + 1e-9*eye(size(S)));

x = x_pred + K*(z - z_hat);
Pk = P_pred - K*S*K';

%% ---------------- Output ----------------
xhat = x;
P = Pk;

end

== matlab function generic_truck/TruckMaker/Tractor_Subsystem /ONE_TRACK_MODEL_TRACTOR_UKF/Included_trailer  ==
  data: z input; u input; xhat output; Q input; R input; Ts input; data input; P output; dxdt output; innovation output; K_out output; S_out output; z_pred_out output
function [xhat, P, dxdt, innovation, K_out, S_out, z_pred_out] = UKF_TruckTrailer(z,u,Q,R,Ts,data)

persistent x Pk dxdt_old t

%% =========================
%% INIT
%% =========================
if isempty(x)
    x = [15;0.1;0.1;7.5;7.5;0;0;6]; % [vx vy wz Cf Cr psi wz_tr Cr_tr]
end

if isempty(Pk)
    Pk = diag([0.1 0.1 0.1 5 5 0.1 0.1 5]);
end

if isempty(dxdt_old)
    dxdt_old = zeros(8,1);
end

if isempty(t)
    t = 0;
end
t = data;

if t < 30
    xhat=x; P=Pk; dxdt=dxdt_old;
    
    innovation=zeros(length(z),1);
    K_out=zeros(length(x), length(z));
    S_out=eye(length(z));
    z_pred_out=zeros(length(z),1);
    return
end

%% =========================
%% CONSTANTS
%% =========================
g = 9.82;

% Truck
m = 6800; Jz = 12994.917; Rwheel = 0.49;

% Trailer
m_tr = 31960; Jz_tr = 145971.764;

% Geometry &  koordinat punkter på Truck
p_cog = [3.473;0;0.925];
p_fax = [4.520;0;0.490];
p_rax = [0.950;0;0.490];
p_imu = [3.600;0;1.000];
hitch = [1.9;0;1.21];

Rcog = p_imu - p_cog;



% Geometry Trailer
p_cog_tr = [-6.195;0;1.95];
p_rax_tr = [-9.0;0;0.490];
hitch_tr = [-1.25;0;1.25];

lf = abs(p_fax(1)-p_cog(1)); 
lr = abs(p_cog(1)-p_rax(1)); 
L = lf + lr;

h = p_cog(3);

Rfax = p_fax - p_cog; Rfax(3)=-p_cog(3);
Rrax = p_rax - p_cog; Rrax(3)=-p_cog(3);

Rhitch = hitch - p_cog;
lhitch = Rhitch(1);

lfhitch = abs(p_fax(1) -hitch(1)); 

lf_tr = abs(hitch_tr(1)-p_cog_tr(1));
lr_tr = abs(p_cog_tr(1)-p_rax_tr(1));
L_tr = lf_tr + lr_tr;
h_tr = p_cog_tr(3);
hHitch= hitch(3);

Rrax_tr = p_rax_tr - hitch_tr; Rrax_tr(3)=-hitch_tr(3);

%% =========================
%% INPUTS
%% =========================
delta = u(1); % steering to raod angle 

% Rear wheel driv
T_rl = u(2);   
T_rr = u(3);

Fxh = u(4); % Inertial Frame  
Fyh = u(5); % Inertial Frame 

Fx_vehicle = (T_rl+T_rr)/Rwheel;

%% =========================
%% UKF PARAMS
%% =========================
n = length(x);
nSPx = 2*n+1;

W0 = 1 - n/3;
Wi = (1 - W0)/(2*n);
gamma = sqrt(n/(1 - W0));

%% =========================
%% SIGMA POINTS (PRIOR)
%% =========================
Pk = (Pk+Pk')/2 + 1e-9*eye(n);
Sx = chol(Pk,'lower');

X_pre = zeros(n,nSPx);
X_pre(:,1) = x;

for i=1:n
    X_pre(:,i+1)   = x + gamma*Sx(:,i);
    X_pre(:,i+1+n) = x - gamma*Sx(:,i);
end

%% =========================
%% PREDICTION
%% =========================
X_pred = zeros(n,nSPx);
dxdt_model = zeros(n,1);

for k=1:nSPx

    Xk = X_pre(:,k);
    % Traktor CoG
    vx=Xk(1); vy=Xk(2); wz=Xk(3);
    Cf=Xk(4); Cr=Xk(5);
    
    %Trialer 
    psi=Xk(6); wz_tr=Xk(7); Cr_tr=Xk(8);

    v_cog=[vx;vy;0];
    omega=[0;0;wz];

    %% ===== TRAILER =====
    v_hitch_truck = v_cog + cross(omega,Rhitch);

    Rot_tr=[cos(psi) -sin(psi) 0;
            sin(psi)  cos(psi) 0;
            0 0 1];

    omega_tr=[0;0;wz_tr];

    v_hitch_trailer = -Rot_tr.' * v_hitch_truck;
    
    % velocity of trailer wheel at rear axle contact point  
    v_tr_ax = v_hitch_trailer + cross(omega_tr,Rrax_tr);
    
    % slip
    alpha_tr = atan2(v_tr_ax(2),max(abs(v_tr_ax(1)),0.1));
    
    % load transfer approximation 
    ax_tr = Fxh/m_tr;
    
    Fz_hitch = m_tr*g*lr_tr/L_tr + m_tr*ax_tr*(h_tr-hHitch)/L_tr;
    Fz_tr    = m_tr*g - Fz_hitch;
    
    %Brush Model 
    Fy_tr = -Cr_tr*alpha_tr*Fz_tr;

    %% ===== TRUCK =====
    %Rotation Matris 
    Rotf=[cos(delta) -sin(delta) 0;
          sin(delta)  cos(delta) 0;
          0                0     1];
    
    % velocities at contact point 
    vf = Rotf.'*(v_cog + cross(omega,Rfax));
    vr = v_cog + cross(omega,Rrax);
    
    %slip per wheel 
    alpha_f = atan2(vf(2),max(abs(vf(1)),0.1));
    alpha_r = atan2(vr(2),max(abs(vr(1)),0.1));
    
    F_hitch_trailer=[u(4);u(5);0];

    F_hitch_body= Rot_tr * F_hitch_trailer;

    % load transfer approximation
    ax_est = (Fx_vehicle + F_hitch_body(1))/m + vy*wz;

    %Ffz = m*g*lr/L - m*ax_est*(h-hHitch)/L + Fz_hitch*(L-lfhitch)/L - F_hitch_body(1)*hHitch/L;
    %Frz = m*g*lf/L + m*ax_est*(h-hHitch)/L;
    
      Ffz = m*g*lr/L + m*ax_est*(h)/L  + Fz_hitch;
      Frz= m*g*lf/L - Ffz ;

    %brsuh model 
    Fy_f = -Cf*alpha_f*Ffz;
    Fy_r = -Cr*alpha_r*Frz;


    %% ===== DYNAMICS =====
    %dvx = (Fx_vehicle - Fy_f*sin(delta) - Fxh*cos(psi) + Fyh*sin(psi))/m + vy*wz;
    dvx = (Fx_vehicle - Fy_f*sin(delta) - F_hitch_body(1))/m + vy*wz;

    %dvy = (Fy_f*cos(delta)+Fy_r - Fyh*cos(psi) - Fxh*sin(psi))/m - vx*wz;
    dvy = (Fy_f*cos(delta) + Fy_r - F_hitch_body(2))/m - vx*wz;
    
    dwz = (lf*Fy_f*cos(delta)-lr*Fy_r)/Jz;% - lhitch*(Fyh*cos(psi) + Fxh*sin(psi)))/Jz;
    %dwz = (lf*Fy_f*cos(delta) -lr*Fy_r - lhitch*(F_hitch_body(2)))/Jz;
    
    dpsi = wz_tr - wz; % Articulation angle 

    dwz_tr = (lr_tr*Fy_tr - lf_tr*Fyh)/Jz_tr;

    if k==1
        dxdt_model=[dvx;dvy;dwz;0;0;dpsi;dwz_tr;0];
    end

    X_pred(:,k) = Xk + Ts*[dvx;
                           dvy;
                           dwz;
                           0;
                           0;
                           dpsi;
                           dwz_tr;
                           0];
end

%% ===== MEAN & COV
x_pred=zeros(n,1);
P_pred=zeros(n);

for k=1:nSPx
    w=(k==1)*W0+(k>1)*Wi;
    x_pred=x_pred+w*X_pred(:,k);
end

for k=1:nSPx
    w=(k==1)*W0+(k>1)*Wi;
    dx=X_pred(:,k)-x_pred;
    P_pred=P_pred+w*(dx*dx');
end

P_pred=P_pred+Q*Ts;
P_pred=(P_pred+P_pred')/2 + 1e-9*eye(n);

%% =========================
%% MEASUREMENT
%% =========================
Sx=chol(P_pred,'lower');

X_post=zeros(n,nSPx);
X_post(:,1)=x_pred;

for i=1:n
    X_post(:,i+1)  =x_pred + gamma*Sx(:,i);
    X_post(:,i+1+n)=x_pred - gamma*Sx(:,i);
end

Z=zeros(length(z),nSPx);

for k=1:nSPx

    Xk=X_post(:,k);

   % Traktor CoG
    vx=Xk(1); vy=Xk(2); wz=Xk(3);
    Cf=Xk(4); Cr=Xk(5);
    
    %Trialer 
    psi=Xk(6); wz_tr=Xk(7); Cr_tr=Xk(8); 
    
    v_cog=[vx;vy;0];
    omega=[0;0;wz];

    %% ===== TRAILER =====
    v_hitch_truck = v_cog + cross(omega,Rhitch);

    Rot_tr=[cos(psi) -sin(psi) 0;
            sin(psi)  cos(psi) 0;
            0 0 1];

    omega_tr=[0;0;wz_tr];

    v_hitch_trailer = Rot_tr.' * v_hitch_truck;
    
    % velocity of trailer wheel at rear axle contact point  
    v_tr_ax = v_hitch_trailer + cross(omega_tr,Rrax_tr);
    
    % slip
    alpha_tr = atan2(v_tr_ax(2),max(abs(v_tr_ax(1)),0.1));
    
    % load transfer approximation 
    ax_tr = (Fxh) / m_tr; % misstänker att vi kan ha ett fel här 
    
    Fz_hitch = m_tr*g*lr_tr/L_tr + m_tr*ax_tr*(h_tr-hHitch)/L_tr;
    Fz_tr = m_tr*g - Fz_hitch;
    
    %Brush Model 
    Fy_tr = -Cr_tr*alpha_tr*Fz_tr;

    %% ===== TRUCK =====    
    %Rotation Matris 
    Rotf=[cos(delta) -sin(delta) 0;
          sin(delta)  cos(delta) 0;
          0                0     1];
    
    % velocities at contact point 
    vf = Rotf.'*(v_cog + cross(omega,Rfax));
    vr = v_cog + cross(omega,Rrax);
    
    %slip per wheel 
    alpha_f = atan2(vf(2),max(abs(vf(1)),0.1));
    alpha_r = atan2(vr(2),max(abs(vr(1)),0.1));
    
    F_hitch_trailer=[u(4);u(5);0];

    F_hitch_body= Rot_tr* F_hitch_trailer;

    % load transfer approximation
    ax_est = (Fx_vehicle + F_hitch_body(1))/m + vy*wz;

    %Ffz = m*g*lr/L - m*ax_est*(h)/L + Fz_hitch*(L-lfhitch)/L - F_hitch_body(1)*hHitch/L;
    %Frz = m*g*lf/L + m*ax_est*(h-hHitch)/L;

      Ffz = m*g*lr/L + m*ax_est*(h)/L  + Fz_hitch;
      Frz= m*g*lf/L - Ffz ;

    %brsuh model 
    Fy_f = -Cf*alpha_f*Ffz;
    Fy_r = -Cr*alpha_r*Frz;


    %% ===== DYNAMICS =====
    %dvx = (Fx_vehicle - Fy_f*sin(delta) - Fxh*cos(psi) + Fyh*sin(psi))/m + vy*wz;
    dvx = (Fx_vehicle - Fy_f*sin(delta) - F_hitch_body(1))/m ;

    %dvy = (Fy_f*cos(delta)+Fy_r - Fyh*cos(psi) - Fxh*sin(psi))/m - vx*wz;
    dvy = (Fy_f*cos(delta)+ Fy_r - F_hitch_body(2))/m;
    
    dwz = (lf*Fy_f*cos(delta)-lr*Fy_r)/Jz;%  - lhitch*(Fyh*cos(psi) + Fxh*sin(psi)))/Jz;
    %dwz = (lf*Fy_f*cos(delta) -lr*Fy_r - lhitch*(F_hitch_body(2)))/Jz;
    
    dpsi = wz_tr - wz; % Articulation angle 

    dwz_tr = (lr_tr*Fy_tr - lf_tr*Fyh )/Jz_tr;

    a_cog=[dvx;dvy;0];
    alpha_vec=[0;0;dwz];

    a_imu=a_cog + cross(omega,cross(omega,Rcog)) + cross(alpha_vec,Rcog);
    v_imu=v_cog + cross(omega,Rcog);

    omega_rl=vx/Rwheel;
    omega_rr=vx/Rwheel;

    omega_tr_ML= v_tr_ax(1)/Rwheel;
    omega_tr_MR= v_tr_ax(1)/Rwheel;

    Z(:,k)=[a_imu(1:2); v_imu(1);v_imu(2); wz; omega_rl; omega_rr; omega_tr_ML; omega_tr_MR];
end

%% ===== REST (sensor selection + update) = DIN ORIGINAL
z_pred=zeros(length(z),1);
for k=1:nSPx
    w=(k==1)*W0+(k>1)*Wi;
    z_pred=z_pred+w*Z(:,k);
end

valid_idx=true(length(z),1);
valid_idx=valid_idx & ~isnan(z);

z_used=z(valid_idx);
z_pred_used=z_pred(valid_idx);
Z_used=Z(valid_idx,:);
R_used=R(valid_idx,valid_idx);

S_cov=zeros(length(z_used));
Pxz=zeros(n,length(z_used));

for k=1:nSPx
    w=(k==1)*W0+(k>1)*Wi;
    dz=Z_used(:,k)-z_pred_used;
    dx=X_post(:,k)-x_pred;
    S_cov=S_cov+w*(dz*dz');
    Pxz=Pxz+w*(dx*dz');
end

S_cov=S_cov+R_used;
S_cov=(S_cov+S_cov')/2 + 1e-9*eye(size(S_cov));

K=Pxz/S_cov;

x=x_pred + K*(z_used - z_pred_used);
Pk=P_pred - K*S_cov*K';
Pk=(Pk+Pk')/2 + 1e-9*eye(n);

%% OUTPUT
xhat=x;
P=Pk;
dxdt=dxdt_model;

innovation=zeros(length(z),1);
innovation(valid_idx)=z_used - z_pred_used;

K_out=zeros(n,length(z));
K_out(:,valid_idx)=K;

S_out=zeros(length(z));
S_out(valid_idx,valid_idx)=S_cov;

z_pred_out=z_pred;

end

== matlab function generic_truck/TruckMaker/Tractor_Subsystem /ONE_TRACK_MODEL_TRACTOR_UKF/MATLAB Function ==
  data: z input; u input; Cf output; Cr output; alpha_f output; alpha_r output
function [Cf, Cr, alpha_f, alpha_r] = stiffness_computation(z, u)
%
% Signal: z = [ ax; ay; az; 
%               vx; vy; vz;
%               rx; ry; rz;
%               alphax; alphay; alphaz;
%               wFL; wFR; wRL; wRR; ]
%
%         u = [ delta; T_rl; T_rr; ]
%

% ------------------------------------------------------------------------%
% Physics
% ------------------------------------------------------------------------%

g = 9.82; % [m/s^2]

% ------------------------------------------------------------------------%
% Truck Parameters
% ------------------------------------------------------------------------%

% Mass [kg]
m = 6800;

% Inertial tensor [kg m^2]
J = [
     5430.025, 0.000,    -589.488;
     0.000,    9407.562,  0.000;
    -589.488,  0.000,     12994.917;
];

% Position vectors [m]
p_cog  = [3.473, 0.000, 0.925].';  % Center of Gravity
p_fax  = [4.520, 0.000, 0.490].';  % Front axle
p_rax  = [0.950, 0.000, 0.490].';  % Rear axle
p_bod  = [3.600, 0.000, 1.000].';  % Body frame
p_imu  = p_bod;

% p_wfl  = [4.520,  1.050, 0.490].'; % Front wheel left
% p_wfr  = [4.520, -1.050, 0.490].'; % Front wheel right
% 
% p_wrl  = [0.950,  1.050, 0.490].'; % Rear wheel left
% p_wrcl = [0.950,  0.860, 0.490].'; % Rear wheel carrier left
% p_wrcr = [0.950, -0.860, 0.490].'; % Rear wheel carrier right
% p_wrr  = [0.950, -1.050, 0.490].'; % Rear wheel right
% 
% Axle load
% m_f = 4805.882; % [kg]
% m_r = 2194.118; % [kg]
% 
% Wheel base
% long = [1,0,0] * abs(p_fax - p_rax); % length [m]
% wide = [0,1,0] * abs(p_wrr - p_wrl); % width  [m]

% CoG hight
high = p_cog(3);

% Wheel radius
% Rwf = 0.505;
% Rwr = 0.505;

% longitudinal distance from cog to axles
lf = [1,0,0] * abs(p_fax - p_cog);
lr = [1,0,0] * abs(p_rax - p_cog);

% ------------------------------------------------------------------------%
% Inputs
% ------------------------------------------------------------------------%

a =  [z(1:2);0]; % IMU acceleration
v =  [z(3:4);0]; % IMU velocity

alpha = [0;0;0];     % IMU yaw acceleration

omega = [0;0;z(end)];  % IMU yaw rate


delta = u(1); % steering angle of one-track front wheel (pre-computed)

T_rl = u(2); % rear left  torque (not used)
T_rr = u(3); % rear right torque (not used)
 
% ------------------------------------------------------------------------%
% Translate measurements
% ------------------------------------------------------------------------%

% displacement vectors
Rfax = p_fax - p_imu; Rfax(3) = -p_imu(3); % straight projection to contact
Rrax = p_rax - p_imu; Rrax(3) = -p_imu(3); % --||--
Rcog = p_cog - p_imu;

% rotation matrix
Rotf = [ 
   cos(delta), -sin(delta), 0;
   sin(delta),  cos(delta), 0;
            0,           0, 1;
];

% velocity translation
% --------------------
vf = Rotf.' * (v + cross(omega, Rfax));
vr = eye(3) * (v + cross(omega, Rrax));

% acceleration translation 
% ------------------------
acog = a + cross(omega, cross(omega, Rcog)) + cross(alpha, Rcog);

% ------------------------------------------------------------------------%
% Computation
% ------------------------------------------------------------------------%

% lateral forces
% --------------
%Ffy = (J(3,3)*alpha(3)+m*acog(2)*lr) / (long * cos(delta));
%Fry = (m*acog(2)*lf - J(3,3)*alpha(3)) / long;

Ffy = (acog(2)*lr) / cos(delta);
Fry = (acog(2)*lf);

% slip
% ----
alpha_f = atan2(vf(2), max(abs(vf(1)), .1));
alpha_r = atan2(vr(2), max(abs(vr(1)), .1));

% normal forces
% -------------
%Ffz = m*g*lr/long - m*acog(1)*high/long;
%Frz = m*g*lf/long + m*acog(1)*high/long;

Ffz = g*lr - acog(1)*high;
Frz = g*lf + acog(1)*high;

% normalized coefficients
% -----------------------
Cf = Ffy / (alpha_f * Ffz); % reference 
Cr = Fry / (alpha_r * Frz); % reference
